simulink model "sat_sim"  (R2021a)
settings: Solver=VariableStepAuto  StartTime=0.0  StopTime=100  RelTol=1e-3
values from neighbouring files (symbols this model uses):
  A = [0 1; 0 0]    [sat.m]
  A_new = [0 1 0; 0 0 1; 0 0 0]    [sat.m]
  B = [0; 1]    [sat.m]
  B_new = [0 1 0]    [sat.m]
  C = [1 0]    [sat.m]
  C_new = [1 0 0]    [sat.m]
  L = place(A',C',p).'    [sat.m]
  L_new = place(A_new', C_new', p_new)    [sat.m]
settings Model: Creator=davidrico  LastModifiedBy=davidrico

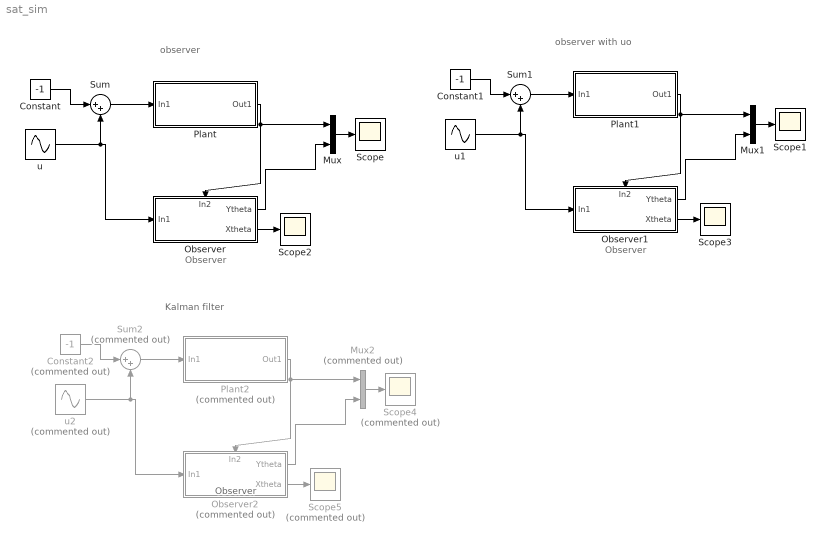
== system sat_sim ==
  note: observer with uo
  note: observer
  note: Observer
  note: Observer
  note: Kalman filter
  note: Observer
  Constant : Constant  Value=-1
  Constant1 : Constant  Value=-1
  Constant2 : Constant  Commented=on  Value=-1
  Mux : Mux  Inputs=2
  Mux1 : Mux  Inputs=2
  Mux2 : Mux  Commented=on  Inputs=2
  Observer : Subsystem
      settings: PortSchema="{\"entries\":[{\"content\":{\"sides\":[{\"content\":{\"connectorIds\":[\"In1\"]},\"type\":\"ConnectorPlacement.EquallySpacedRectSide\",\"uuid\":\"c649fa55-f2dd-4471-a628-d4e2ecd70080\"},{\"content\":{\"connectorIds\":[\"Out1\",\"Out2\"],\"side\":\"RIGHT\"},\"type\":\"ConnectorPlacement.EquallySpacedRectSide\",\"uuid\":\"740a641d-8c10-427a-b208-edf66c3f49d4\"},{\"content\":{\"connectorIds\":[\"In2\"],\"side\":\"TOP\"},\"type\":\"ConnectorPlacement.EquallySpacedRectSide\",\"uuid\":\"5c9efc11-8b85-444c-9a35-938e2dea4a09\"}]},\"type\":\"ConnectorPlacement.EquallySpacedConnector\",\"uuid\":\"0b76e225-6789-4662-943a-1350fe577cbc\"}],\"packageUris\":[\"http://schema.mathworks.com/mf0/Connector/R2020b\"],\"version\":\"1.0\"}"
  Observer1 : Subsystem
      settings: PortSchema="{\"entries\":[{\"content\":{\"sides\":[{\"content\":{\"connectorIds\":[\"In1\"]},\"type\":\"ConnectorPlacement.EquallySpacedRectSide\",\"uuid\":\"c649fa55-f2dd-4471-a628-d4e2ecd70080\"},{\"content\":{\"connectorIds\":[\"Out1\",\"Out2\"],\"side\":\"RIGHT\"},\"type\":\"ConnectorPlacement.EquallySpacedRectSide\",\"uuid\":\"740a641d-8c10-427a-b208-edf66c3f49d4\"},{\"content\":{\"connectorIds\":[\"In2\"],\"side\":\"TOP\"},\"type\":\"ConnectorPlacement.EquallySpacedRectSide\",\"uuid\":\"5c9efc11-8b85-444c-9a35-938e2dea4a09\"}]},\"type\":\"ConnectorPlacement.EquallySpacedConnector\",\"uuid\":\"0b76e225-6789-4662-943a-1350fe577cbc\"}],\"packageUris\":[\"http://schema.mathworks.com/mf0/Connector/R2020b\"],\"version\":\"1.0\"}"
  Observer2 : Subsystem  Commented=on
      settings: PortSchema="{\"entries\":[{\"content\":{\"sides\":[{\"content\":{\"connectorIds\":[\"In1\"]},\"type\":\"ConnectorPlacement.EquallySpacedRectSide\",\"uuid\":\"c649fa55-f2dd-4471-a628-d4e2ecd70080\"},{\"content\":{\"connectorIds\":[\"Out1\",\"Out2\"],\"side\":\"RIGHT\"},\"type\":\"ConnectorPlacement.EquallySpacedRectSide\",\"uuid\":\"740a641d-8c10-427a-b208-edf66c3f49d4\"},{\"content\":{\"connectorIds\":[\"In2\"],\"side\":\"TOP\"},\"type\":\"ConnectorPlacement.EquallySpacedRectSide\",\"uuid\":\"5c9efc11-8b85-444c-9a35-938e2dea4a09\"}]},\"type\":\"ConnectorPlacement.EquallySpacedConnector\",\"uuid\":\"0b76e225-6789-4662-943a-1350fe577cbc\"}],\"packageUris\":[\"http://schema.mathworks.com/mf0/Connector/R2020b\"],\"version\":\"1.0\"}"
  Plant : Subsystem
  Plant1 : Subsystem
  Plant2 : Subsystem  Commented=on
  Scope{,1..3} (4 alike) : Scope
  Scope4 : Scope  Commented=on
  Scope5 : Scope  Commented=on
  Sum : Sum  Inputs=|++
  Sum1 : Sum  Inputs=|++
  Sum2 : Sum  Commented=on  Inputs=|++
  u : Sin  SampleTime=0
  u1 : Sin  SampleTime=0
  u2 : Sin  Commented=on  SampleTime=0
  wires:
  Plant/1(Out1) -> Observer/2(In2), Mux/1
  Observer/1(Ytheta) -> Mux/2
  Observer/2(Xtheta) -> Scope2/1
  u/1 -> Sum/2, Observer/1(In1)
  Mux/1 -> Scope/1
  Constant/1 -> Sum/1
  Sum/1 -> Plant/1(In1)
  Mux1/1 -> Scope1/1
  u1/1 -> Sum1/2, Observer1/1(In1)
  Observer1/1(Ytheta) -> Mux1/2
  Observer1/2(Xtheta) -> Scope3/1
  Plant1/1(Out1) -> Observer1/2(In2), Mux1/1
  Constant1/1 -> Sum1/1
  Sum1/1 -> Plant1/1(In1)
  u2/1 -> Sum2/2, Observer2/1(In1)
  Constant2/1 -> Sum2/1
  Plant2/1(Out1) -> Observer2/2(In2), Mux2/1
  Observer2/1(Ytheta) -> Mux2/2
  Mux2/1 -> Scope4/1
  Observer2/2(Xtheta) -> Scope5/1
  Sum2/1 -> Plant2/1(In1)

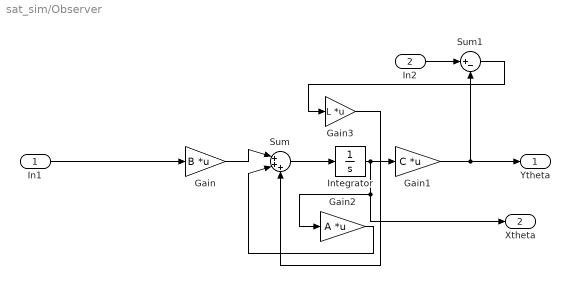
== system sat_sim/Observer ==
  In1 : Inport
  In2 : Inport  Port=2
  Gain : Gain  Gain=B  Multiplication=Matrix(K*u) (u vector)
  Gain1 : Gain  Gain=C  Multiplication=Matrix(K*u) (u vector)
  Gain2 : Gain  Gain=A  Multiplication=Matrix(K*u) (u vector)
  Gain3 : Gain  Gain=L  Multiplication=Matrix(K*u)
  Integrator : Integrator  InitialCondition=[0; 0]
  Sum : Sum  Inputs=|+++
  Sum1 : Sum  Inputs=|+-
  Ytheta : Outport
  Xtheta : Outport  Port=2
  wires:
  Gain/1 -> Sum/1
  Gain2/1 -> Sum/2
  In1/1 -> Gain/1
  Integrator/1 -> Xtheta/1, Gain2/1, Gain1/1
  Gain1/1 -> Sum1/2, Ytheta/1
  Sum/1 -> Integrator/1
  In2/1 -> Sum1/1
  Sum1/1 -> Gain3/1
  Gain3/1 -> Sum/3

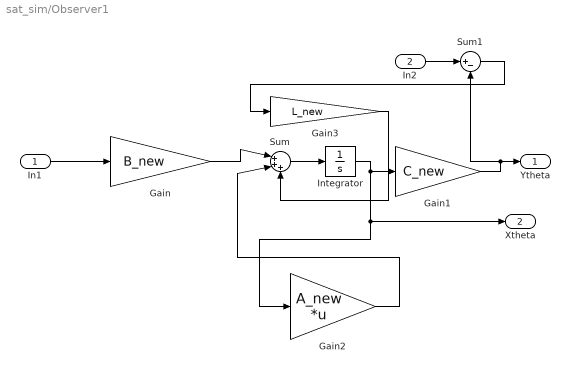
== system sat_sim/Observer1 ==
  In1 : Inport
  In2 : Inport  Port=2
  Gain : Gain  Gain=B_new
  Gain1 : Gain  Gain=C_new
  Gain2 : Gain  Gain=A_new  Multiplication=Matrix(K*u) (u vector)
  Gain3 : Gain  Gain=L_new
  Integrator : Integrator  InitialCondition=[0; 0; 0]
  Sum : Sum  Inputs=|+++
  Sum1 : Sum  Inputs=|+-
  Ytheta : Outport
  Xtheta : Outport  Port=2
  wires:
  Gain/1 -> Sum/1
  Gain2/1 -> Sum/2
  In1/1 -> Gain/1
  Integrator/1 -> Xtheta/1, Gain2/1, Gain1/1
  Gain1/1 -> Sum1/2, Ytheta/1
  Sum/1 -> Integrator/1
  In2/1 -> Sum1/1
  Sum1/1 -> Gain3/1
  Gain3/1 -> Sum/3

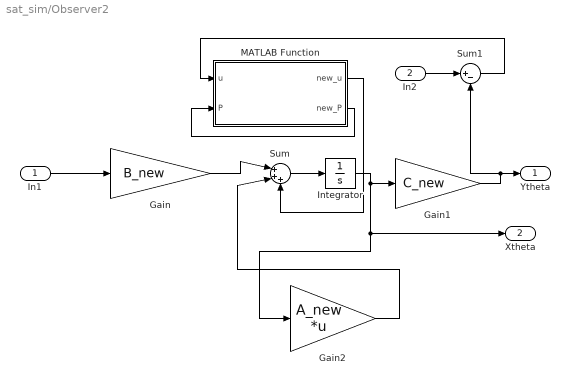
== system sat_sim/Observer2 ==
  In1 : Inport
  In2 : Inport  Port=2
  Gain : Gain  Gain=B_new
  Gain1 : Gain  Gain=C_new
  Gain2 : Gain  Gain=A_new  Multiplication=Matrix(K*u) (u vector)
  Integrator : Integrator  InitialCondition=[0; 0; 0]
  MATLAB Function : MATLAB Function  TreatAsAtomicUnit=on
  Sum : Sum  Inputs=|+++
  Sum1 : Sum  Inputs=|+-
  Ytheta : Outport
  Xtheta : Outport  Port=2
  wires:
  Gain/1 -> Sum/1
  Gain2/1 -> Sum/2
  In1/1 -> Gain/1
  Integrator/1 -> Xtheta/1, Gain2/1, Gain1/1
  Gain1/1 -> Sum1/2, Ytheta/1
  Sum/1 -> Integrator/1
  In2/1 -> Sum1/1
  Sum1/1 -> MATLAB Function/1(u)
  MATLAB Function/1(new_u) -> Sum/3
  MATLAB Function/2(new_P) -> MATLAB Function/2(P)

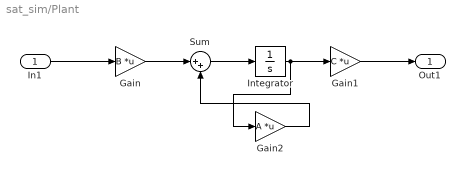
== system sat_sim/Plant ==
  In1 : Inport
  Gain : Gain  Gain=B  Multiplication=Matrix(K*u) (u vector)
  Gain1 : Gain  Gain=C  Multiplication=Matrix(K*u) (u vector)
  Gain2 : Gain  Gain=A  Multiplication=Matrix(K*u) (u vector)
  Integrator : Integrator  InitialCondition=[10; 10]
  Sum : Sum  Inputs=|++
  Out1 : Outport
  wires:
  In1/1 -> Gain/1
  Gain/1 -> Sum/1
  Sum/1 -> Integrator/1
  Integrator/1 -> Gain2/1, Gain1/1
  Gain1/1 -> Out1/1
  Gain2/1 -> Sum/2

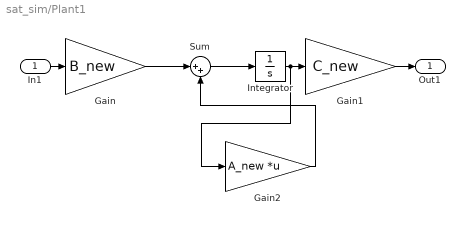
== system sat_sim/Plant1 ==
  In1 : Inport
  Gain : Gain  Gain=B_new
  Gain1 : Gain  Gain=C_new
  Gain2 : Gain  Gain=A_new  Multiplication=Matrix(K*u) (u vector)
  Integrator : Integrator  InitialCondition=[10; 10; 10]
  Sum : Sum  Inputs=|++
  Out1 : Outport
  wires:
  In1/1 -> Gain/1
  Gain/1 -> Sum/1
  Sum/1 -> Integrator/1
  Integrator/1 -> Gain2/1, Gain1/1
  Gain1/1 -> Out1/1
  Gain2/1 -> Sum/2

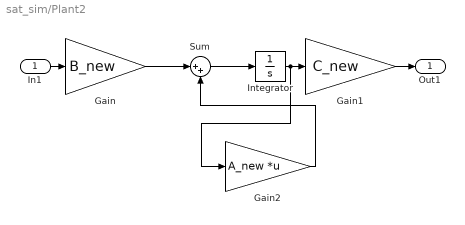
== system sat_sim/Plant2 ==
  In1 : Inport
  Gain : Gain  Gain=B_new
  Gain1 : Gain  Gain=C_new
  Gain2 : Gain  Gain=A_new  Multiplication=Matrix(K*u) (u vector)
  Integrator : Integrator  InitialCondition=[10; 10; 10]
  Sum : Sum  Inputs=|++
  Out1 : Outport
  wires:
  In1/1 -> Gain/1
  Gain/1 -> Sum/1
  Sum/1 -> Integrator/1
  Integrator/1 -> Gain2/1, Gain1/1
  Gain1/1 -> Out1/1
  Gain2/1 -> Sum/2

== matlab function sat_sim/Observer2/MATLAB Function ==
  data: u input; new_u output; P input; new_P output
function [new_u, new_P] = fcn(u, P)
A = [0 1 0; 0 0 1; 0 0 0];
B = [0 1 0];
C = [1 0 0];

Q = C'*C;
R = B*B';
new_P = A*P + P*A' - P*C'*inv(R)*C*P + Q;
L = P*C'*inv(R);
new_u = L.*u;
